simulink model "dac_test"  (R2024a)
settings: Solver=FixedStepAuto  StartTime=0.0  StopTime=Inf  RelTol=1e-3  EnableMultiTasking=on
libraries: c2802xlib x1, c2837xDlib x1
settings Model: ExtModeTrigDuration=8  Creator=Dell  LastModifiedBy=Dell
settings OptimizationCC: DefaultUnderspecifiedDataType=single  EnhancedBackFolding=on  PassReuseOutputArgsAs=Individual arguments  MaxStackSize=1024  OptimizeBlockOrder=speed  DifferentSizesBufferReuse=on  OptimizationCustomize=off  EfficientTunableParamExpr=on
settings DebuggingCC: ParameterTunabilityLossMsg=error
settings HardwareCC: ProdBitPerChar=16  ProdBitPerInt=16  ProdBitPerPointer=32  ProdBitPerSizeT=32  ProdBitPerPtrDiffT=32  ProdLargestAtomicInteger=Integer  ProdLargestAtomicFloat=None  ProdWordSize=16  ProdLongLongMode=on  ProdHWDeviceType=Texas Instruments->C2000  HardwareBoardFeatureSet=SoCBlockset
settings SFSimCC: MATLABDynamicMemAlloc=off
settings RTWCC: Description=Embedded Coder  SystemTargetFile=ert.tlc  HardwareBoard=TI Piccolo F280049C LaunchPad  TemplateMakefile=ert_default_tmf  Toolchain=Texas Instruments Code Composer Studio (C2000)  CodeProfilingSaveOptions=MetricsOnly
settings CodeAppCC: ForceParamTrailComments=on  IgnoreCustomStorageClasses=off  OperatorAnnotations=on  SimulinkDataObjDesc=on  SFDataObjDesc=on  InsertBlockDesc=on
settings ERTTargetCC: CodeReplacementLibrary=TI C28x  ExtModeTransport=4  ExtModeStaticAlloc=on  ExtModeAutomaticAllocSize=off  ExtModeStaticAllocSize=5000  ExtModeMexFile=ext_xcp  ExtModeIntrfLevel=Level2 - Open

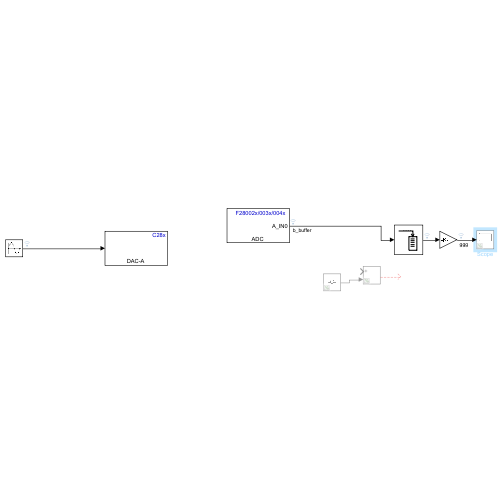
[thumbnail: Simulink's stored preview of the top-level diagram]
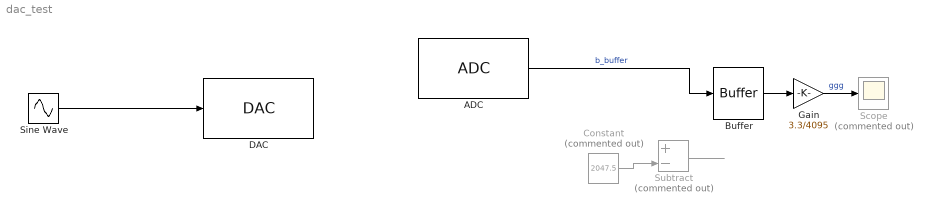
== system dac_test ==
  ADC : c2802xlib/ADC  blkParamProc=C2000_Type5  ADCModule=A  samplingMode=Single sample mode  ADCResolution=12-bit (Single-ended input)  useSOC1=SOC0  useSOC2=SOC0_SOC1  SOCAcquisitionWindow=8  SOCTriggerSource=Software  SOCInterruptTrigger=No ADCINT  Ts=1e-6  dType=uint16  postInterrupt=off  interruptSel=ADCINT1  ADCINTContinuous=on  endma=off  chdma=1  conv1=ADCINA0  conv2=ADCINA0 and ADCINB0  conv1_Type4=ADCIN0  conv2_Type4=ADCIN0 and ADCIN1
      settings: LibrarySourceBlock=c28004xlib/ADC
  Buffer : Buffer  OutputFrames=off
  Constant : Constant  Commented=on  Value=2047.5  OutDataTypeStr=single
  DAC : c2837xDlib/DAC  channel=A  saturate=off
      settings: LibrarySourceBlock=c28004xlib/DAC
  Gain : Gain  Gain=3.3/4095
  Scope : Scope  Commented=on
  Sine Wave : Sin  SineType=Sample based  Amplitude=2047.5  Bias=2047.5  SampleTime=0.01
  Subtract : Sum  Commented=on  Inputs=+-
  wires:
  Sine Wave/1 -> DAC/1
  Buffer/1 -> Gain/1
  Gain/1 -> Scope/1  "ggg"
  ADC/1 -> Buffer/1  "b_buffer"
  Subtract/1 -> ?
  Constant/1 -> Subtract/2
